simulink model "c00010M_harness"  (R2018a)
settings: Solver=ode3  StartTime=0.0  StopTime=10.0  RelTol=1e-3  EnableMultiTasking=on
undefined symbols (not defined in the file): b, DiscIntNeverNeededParam, J, K, L, PosMinimaW3, R, sigbuilder_block
(part 1 of 4)
settings Model: Creator=aarrieta  LastModifiedBy=umarkiegi
settings DataIOCC: LimitDataPoints=on  SaveFormat=Array
settings OptimizationCC: LifeSpan=inf
settings DebuggingCC: UnderspecifiedInitializationDetection=Classic  MergeDetectMultiDrivingBlocksExec=none  SolverPrmCheckMsg=warning  StateNameClashWarn=warning  SFUnexpectedBacktrackingDiag=warning  SFNoUnconditionalDefaultTransitionDiag=warning  SFExecutionAtInitializationDiag=none
settings HardwareCC: ProdBitPerPointer=32  ProdBitPerSizeT=32  ProdBitPerPtrDiffT=32  ProdLargestAtomicFloat=None  ProdIntDivRoundTo=Undefined  ProdEndianess=Unspecified  ProdWordSize=32  ProdHWDeviceType=32-bit Generic
settings ModelReferenceCC: PropagateSignalLabelsOutOfModel=off
settings CodeAppCC: StateflowObjectComments=on
settings GRTTargetCC: TargetLangStandard=C89/C90 (ANSI)  GeneratePreprocessorConditionals=Disable all
settings ConfigComp: CovMetricSettings=dw  CovHtmlReporting=on  CovSaveCumulativeToWorkspaceVar=on  CovSaveSingleToWorkspaceVar=on  CovExternalEMLEnable=off  DVMaxTestCaseSteps=20  DVTestSuiteOptimization=CombinedObjectives (Nonlinear Extended)  DVDetectFloatOverflow=off

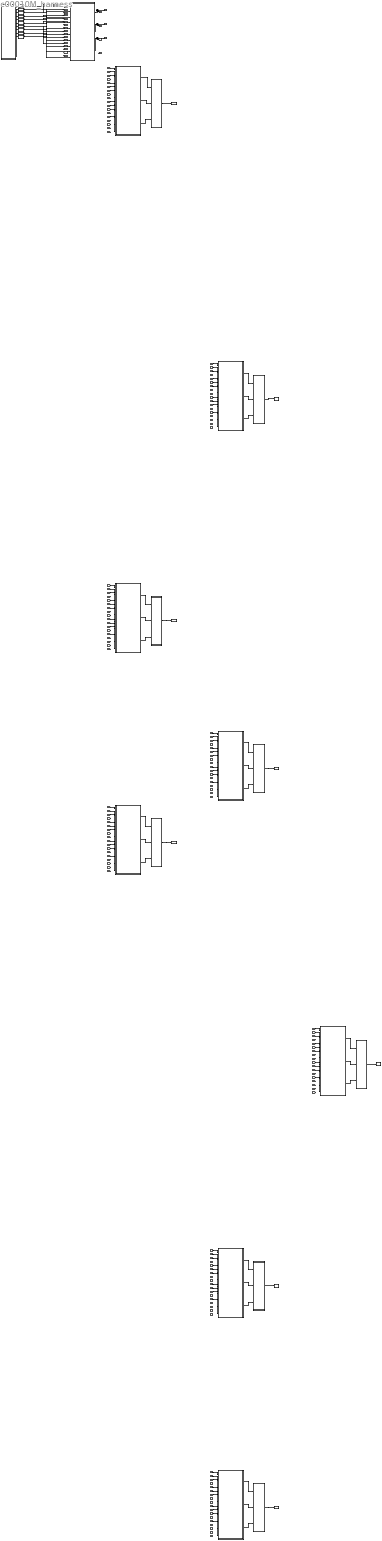
== system c00010M_harness ==
  CPSUT : Subsystem
  Eval : Subsystem
  Eval10 : Subsystem
  Eval24 : Subsystem
  Eval29 : Subsystem
  Eval36 : Subsystem
  Eval39 : Subsystem
  Eval53 : Subsystem
  Eval7 : Subsystem
  Inputs : Subsystem  Tag=STV Subsys  LoadFcn=sigbuilder_block('load');  StartFcn=sigbuilder_block('start');  StopFcn=sigbuilder_block('stop');  ClipboardFcn=sigbuilder_block('clipboard');  mask(Sigbuilder block){tuvar=[0:10]}
      mask init:
      | if ~strcmp(get_param(bdroot(gcb),'SimulationStatus'),'stopped'),tuvar = sigbuilder_block('maskInit'); end
      settings: CopyFcn=sigbuilder_block('copy');  DeleteFcn=sigbuilder_block('delete');  ModelCloseFcn=sigbuilder_block('modelClose');  PreSaveFcn=sigbuilder_block('preSave');  PauseFcn=sigbuilder_block('pause');  ContinueFcn=sigbuilder_block('continue');  NameChangeFcn=sigbuilder_block('namechange');  OpenFcn=sigbuilder_block('open');  CloseFcn=sigbuilder_block('close');
      mask Display: plot(0, 0, 100, 100,[2, 2, 32, 32, 2], [68, 8, 8, 68, 68],[32, 2], [38, 38], [32, 19, 2],[53, 60, 44], [32, 17, 17, 2],[16, 16, 31, 31]);txt = getActiveGroup(gcbh);text(2, 100, txt,'verticalAlignment', 'top');
  M001 : Subsystem
  M008 : Subsystem
  M011 : Subsystem
  M025 : Subsystem
  M030 : Subsystem
  M037 : Subsystem
  M040 : Subsystem
  M054 : Subsystem
  To Workspace : ToWorkspace  VariableName=mutant001  SampleTime=-1
  To Workspace10 : ToWorkspace  VariableName=mutant011  SampleTime=-1
  To Workspace24 : ToWorkspace  VariableName=mutant025  SampleTime=-1
  To Workspace29 : ToWorkspace  VariableName=mutant030  SampleTime=-1
  To Workspace36 : ToWorkspace  VariableName=mutant037  SampleTime=-1
  To Workspace39 : ToWorkspace  VariableName=mutant040  SampleTime=-1
  To Workspace53 : ToWorkspace  VariableName=mutant054  SampleTime=-1
  To Workspace7 : ToWorkspace  VariableName=mutant008  SampleTime=-1
  dtc_DW1 : DataTypeConversion
  dtc_DW2 : DataTypeConversion
  dtc_DW3 : DataTypeConversion
  dtc_LD : DataTypeConversion
  dtc_O1 : DataTypeConversion
  dtc_O2 : DataTypeConversion
  dtc_O3 : DataTypeConversion
  dtc_P1W2 : DataTypeConversion
  dtc_P1W3 : DataTypeConversion
  dtc_P2W3 : DataTypeConversion
  W1Pos : Outport
  W2Pos : Outport  Port=2
  W3Pos : Outport  Port=3
  tag scope: out1=global, out2=global, out3=global, out4=global
  wires:
  CPSUT/2(W2Pos) -> [out2], W2Pos/1
  CPSUT/3(W3Pos) -> W3Pos/1, [out3]
  [in1] -> M001/1(DW1)
  [in2] -> M001/2(DW2)
  [in3] -> M001/3(DW3)
  [in5] -> M001/4(P1W2)
  [in6] -> M001/5(P2W3)
  [in7] -> M001/6(P1W3)
  [in10] -> M001/7(O1)
  [in11] -> M001/8(O2)
  [in12] -> M001/9(O3)
  [in14] -> M001/10(LD)
  CPSUT/1(W1Pos) -> [out1], W1Pos/1
  M001/1(W1Pos) -> Eval/1(In1)
  M001/2(W2Pos) -> Eval/2(In2)
  M001/3(W3Pos) -> Eval/3(In3)
  Eval/1(Out1) -> To Workspace/1
  [in1] -> M008/1(DW1)
  [in2] -> M008/2(DW2)
  [in3] -> M008/3(DW3)
  [in5] -> M008/4(P1W2)
  [in6] -> M008/5(P2W3)
  [in7] -> M008/6(P1W3)
  [in10] -> M008/7(O1)
  [in11] -> M008/8(O2)
  [in12] -> M008/9(O3)
  [in14] -> M008/10(LD)
  M008/1(W1Pos) -> Eval7/1(In1)
  M008/2(W2Pos) -> Eval7/2(In2)
  M008/3(W3Pos) -> Eval7/3(In3)
  Eval7/1(Out1) -> To Workspace7/1
  [in1] -> M011/1(DW1)
  [in2] -> M011/2(DW2)
  [in3] -> M011/3(DW3)
  [in5] -> M011/4(P1W2)
  [in6] -> M011/5(P2W3)
  [in7] -> M011/6(P1W3)
  [in10] -> M011/7(O1)
  [in11] -> M011/8(O2)
  [in12] -> M011/9(O3)
  [in14] -> M011/10(LD)
  M011/1(W1Pos) -> Eval10/1(In1)
  M011/2(W2Pos) -> Eval10/2(In2)
  M011/3(W3Pos) -> Eval10/3(In3)
  Eval10/1(Out1) -> To Workspace10/1
  [in1] -> M025/1(DW1)
  [in2] -> M025/2(DW2)
  [in3] -> M025/3(DW3)
  [in5] -> M025/4(P1W2)
  [in6] -> M025/5(P2W3)
  [in7] -> M025/6(P1W3)
  [in10] -> M025/7(O1)
  [in11] -> M025/8(O2)
  [in12] -> M025/9(O3)
  [in14] -> M025/10(LD)
  M025/1(W1Pos) -> Eval24/1(In1)
  M025/2(W2Pos) -> Eval24/2(In2)
  M025/3(W3Pos) -> Eval24/3(In3)
  Eval24/1(Out1) -> To Workspace24/1
  [in1] -> M030/1(DW1)
  [in2] -> M030/2(DW2)
  [in3] -> M030/3(DW3)
  [in5] -> M030/4(P1W2)
  [in6] -> M030/5(P2W3)
  [in7] -> M030/6(P1W3)
  [in10] -> M030/7(O1)
  [in11] -> M030/8(O2)
  [in12] -> M030/9(O3)
  [in14] -> M030/10(LD)
  M030/1(W1Pos) -> Eval29/1(In1)
  M030/2(W2Pos) -> Eval29/2(In2)
  M030/3(W3Pos) -> Eval29/3(In3)
  Eval29/1(Out1) -> To Workspace29/1
  [in1] -> M037/1(DW1)
  [in2] -> M037/2(DW2)
  [in3] -> M037/3(DW3)
  [in5] -> M037/4(P1W2)
  [in6] -> M037/5(P2W3)
  [in7] -> M037/6(P1W3)
  [in10] -> M037/7(O1)
  [in11] -> M037/8(O2)
  [in12] -> M037/9(O3)
  [in14] -> M037/10(LD)
  M037/1(W1Pos) -> Eval36/1(In1)
  M037/2(W2Pos) -> Eval36/2(In2)
  M037/3(W3Pos) -> Eval36/3(In3)
  Eval36/1(Out1) -> To Workspace36/1
  [in1] -> M040/1(DW1)
  [in2] -> M040/2(DW2)
  [in3] -> M040/3(DW3)
  [in5] -> M040/4(P1W2)
  [in6] -> M040/5(P2W3)
  [in7] -> M040/6(P1W3)
  [in10] -> M040/7(O1)
  [in11] -> M040/8(O2)
  [in12] -> M040/9(O3)
  [in14] -> M040/10(LD)
  M040/1(W1Pos) -> Eval39/1(In1)
  M040/2(W2Pos) -> Eval39/2(In2)
  M040/3(W3Pos) -> Eval39/3(In3)
  Eval39/1(Out1) -> To Workspace39/1
  [in1] -> M054/1(DW1)
  [in2] -> M054/2(DW2)
  [in3] -> M054/3(DW3)
  [in5] -> M054/4(P1W2)
  [in6] -> M054/5(P2W3)
  [in7] -> M054/6(P1W3)
  [in10] -> M054/7(O1)
  [in11] -> M054/8(O2)
  [in12] -> M054/9(O3)
  [in14] -> M054/10(LD)
  M054/1(W1Pos) -> Eval53/1(In1)
  M054/2(W2Pos) -> Eval53/2(In2)
  M054/3(W3Pos) -> Eval53/3(In3)
  Eval53/1(Out1) -> To Workspace53/1
  Inputs/1(DW1) -> dtc_DW1/1
  dtc_DW1/1 -> CPSUT/1(DW1), [in1]
  Inputs/2(DW2) -> dtc_DW2/1
  dtc_DW2/1 -> CPSUT/2(DW2), [in2]
  Inputs/3(DW3) -> dtc_DW3/1
  dtc_DW3/1 -> CPSUT/3(DW3), [in3]
  Inputs/4(P1W2) -> dtc_P1W2/1
  dtc_P1W2/1 -> CPSUT/4(P1W2), [in5]
  Inputs/5(P2W3) -> dtc_P2W3/1
  dtc_P2W3/1 -> CPSUT/5(P2W3), [in6]
  Inputs/6(P1W3) -> dtc_P1W3/1
  dtc_P1W3/1 -> CPSUT/6(P1W3), [in7]
  Inputs/7(O1) -> dtc_O1/1
  dtc_O1/1 -> CPSUT/7(O1), [in10]
  Inputs/8(O2) -> dtc_O2/1
  dtc_O2/1 -> CPSUT/8(O2), [in11]
  Inputs/9(O3) -> dtc_O3/1
  dtc_O3/1 -> CPSUT/9(O3), [in12]
  Inputs/10(LD) -> dtc_LD/1
  dtc_LD/1 -> CPSUT/10(LD), [in14]

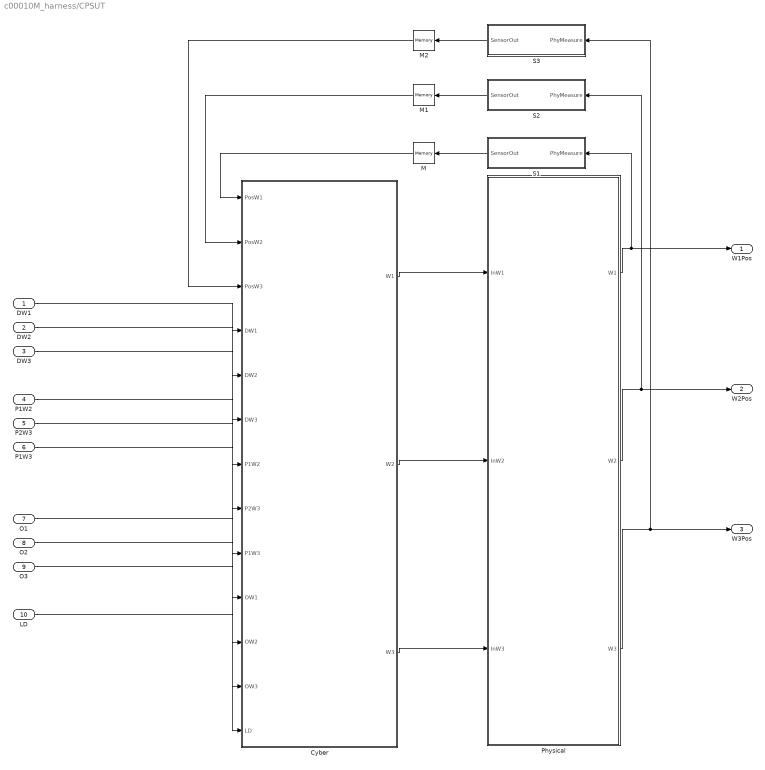
== system c00010M_harness/CPSUT ==
  DW1 : Inport  OutMin=0  OutMax=4  OutDataTypeStr=int8
  DW2 : Inport  Port=2  OutMin=0  OutMax=4  OutDataTypeStr=int8
  DW3 : Inport  Port=3  OutMin=0  OutMax=4  OutDataTypeStr=int8
  P1W2 : Inport  Port=4  OutMin=0  OutMax=4  OutDataTypeStr=int8
  P2W3 : Inport  Port=5  OutMin=0  OutMax=4  OutDataTypeStr=int8
  P1W3 : Inport  Port=6  OutMin=0  OutMax=4  OutDataTypeStr=int8
  O1 : Inport  Port=7  OutDataTypeStr=boolean
  O2 : Inport  Port=8  OutDataTypeStr=boolean
  O3 : Inport  Port=9  OutDataTypeStr=boolean
  LD : Inport  Port=10  OutDataTypeStr=boolean
  Cyber : Subsystem
  M : Memory
  M1 : Memory
  M2 : Memory
  Physical : Subsystem
  S1 : Subsystem
  S2 : Subsystem
  S3 : Subsystem
  W1Pos : Outport
  W2Pos : Outport  Port=2
  W3Pos : Outport  Port=3
  wires:
  P2W3/1 -> Cyber/8(P2W3)
  S1/1(SensorOut) -> M/1
  Physical/1(W1) -> W1Pos/1, S1/1(PhyMeasure)
  S3/1(SensorOut) -> M2/1
  O2/1 -> Cyber/11(OW2)
  Cyber/3(W3) -> Physical/3(InW3)
  LD/1 -> Cyber/13(LD)
  O1/1 -> Cyber/10(OW1)
  Cyber/1(W1) -> Physical/1(InW1)
  Cyber/2(W2) -> Physical/2(InW2)
  M2/1 -> Cyber/3(PosW3)
  P1W2/1 -> Cyber/7(P1W2)
  O3/1 -> Cyber/12(OW3)
  P1W3/1 -> Cyber/9(P1W3)
  DW3/1 -> Cyber/6(DW3)
  M1/1 -> Cyber/2(PosW2)
  Physical/3(W3) -> W3Pos/1, S3/1(PhyMeasure)
  M/1 -> Cyber/1(PosW1)
  DW1/1 -> Cyber/4(DW1)
  Physical/2(W2) -> W2Pos/1, S2/1(PhyMeasure)
  S2/1(SensorOut) -> M1/1
  DW2/1 -> Cyber/5(DW2)

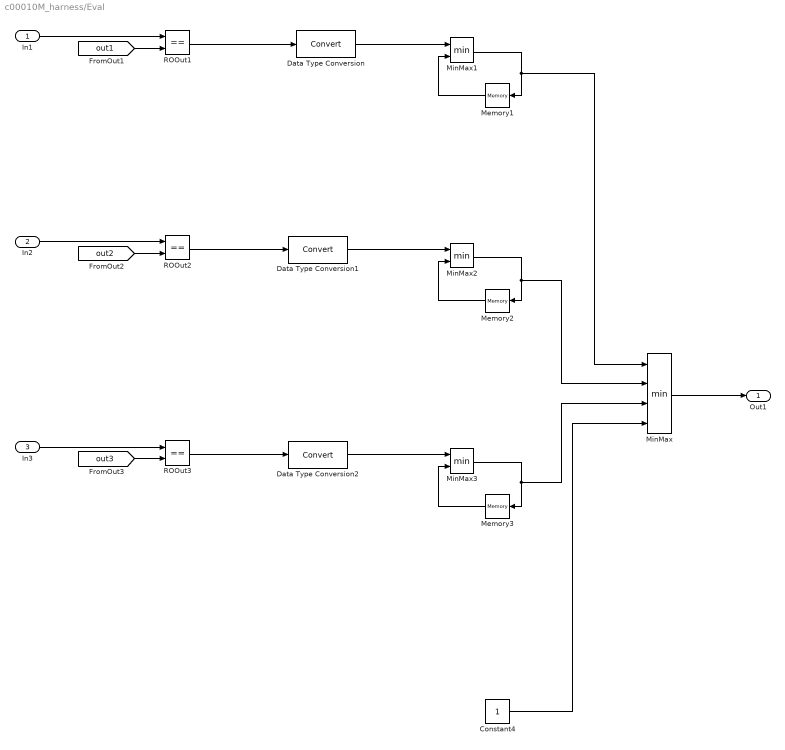
== system c00010M_harness/Eval ==
  In1 : Inport
  In2 : Inport  Port=2
  In3 : Inport  Port=3
  Constant4 : Constant
  Data Type Conversion : DataTypeConversion
  Data Type Conversion1 : DataTypeConversion
  Data Type Conversion2 : DataTypeConversion
  Memory1 : Memory  InitialCondition=1
  Memory2 : Memory  InitialCondition=1
  Memory3 : Memory  InitialCondition=1
  MinMax : MinMax  Inputs=4
  MinMax1 : MinMax  Inputs=2
  MinMax2 : MinMax  Inputs=2
  MinMax3 : MinMax  Inputs=2
  ROOut1 : RelationalOperator  Operator===  OutDataTypeStr=boolean  RndMeth=Simplest
  ROOut2 : RelationalOperator  Operator===  OutDataTypeStr=boolean  RndMeth=Simplest
  ROOut3 : RelationalOperator  Operator===  OutDataTypeStr=boolean  RndMeth=Simplest
  Out1 : Outport
  wires:
  MinMax/1 -> Out1/1
  [out3] -> ROOut3/2
  In3/1 -> ROOut3/1
  [out1] -> ROOut1/2
  In2/1 -> ROOut2/1
  In1/1 -> ROOut1/1
  [out2] -> ROOut2/2
  Memory1/1 -> MinMax1/2
  MinMax3/1 -> MinMax/3, Memory3/1
  ROOut3/1 -> Data Type Conversion2/1
  ROOut2/1 -> Data Type Conversion1/1
  Memory3/1 -> MinMax3/2
  Memory2/1 -> MinMax2/2
  ROOut1/1 -> Data Type Conversion/1
  MinMax2/1 -> MinMax/2, Memory2/1
  MinMax1/1 -> MinMax/1, Memory1/1
  Data Type Conversion/1 -> MinMax1/1
  Data Type Conversion1/1 -> MinMax2/1
  Data Type Conversion2/1 -> MinMax3/1
  Constant4/1 -> MinMax/4

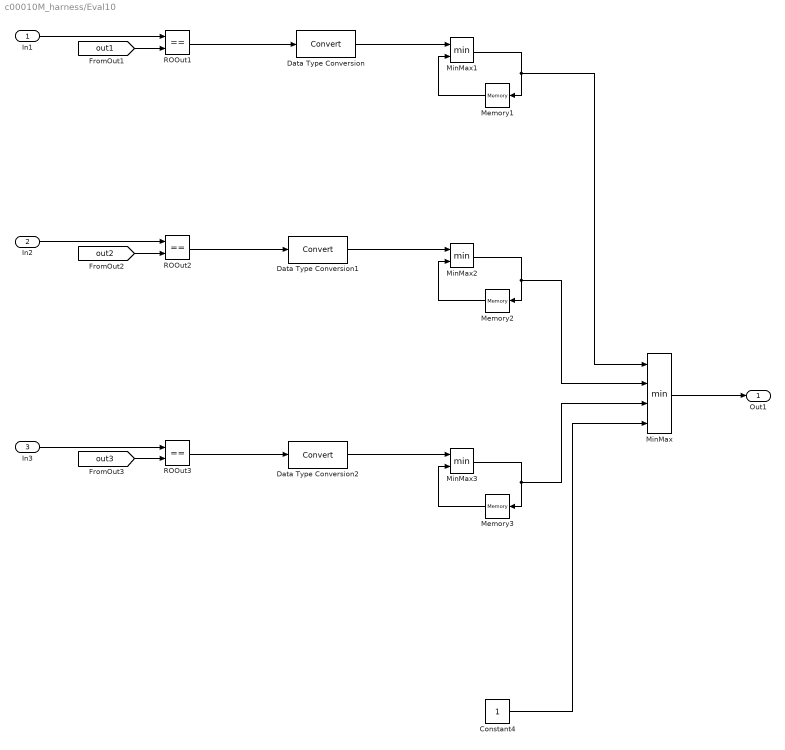
== system c00010M_harness/Eval10 ==
  In1 : Inport
  In2 : Inport  Port=2
  In3 : Inport  Port=3
  Constant4 : Constant
  Data Type Conversion : DataTypeConversion
  Data Type Conversion1 : DataTypeConversion
  Data Type Conversion2 : DataTypeConversion
  Memory1 : Memory  InitialCondition=1
  Memory2 : Memory  InitialCondition=1
  Memory3 : Memory  InitialCondition=1
  MinMax : MinMax  Inputs=4
  MinMax1 : MinMax  Inputs=2
  MinMax2 : MinMax  Inputs=2
  MinMax3 : MinMax  Inputs=2
  ROOut1 : RelationalOperator  Operator===  OutDataTypeStr=boolean  RndMeth=Simplest
  ROOut2 : RelationalOperator  Operator===  OutDataTypeStr=boolean  RndMeth=Simplest
  ROOut3 : RelationalOperator  Operator===  OutDataTypeStr=boolean  RndMeth=Simplest
  Out1 : Outport
  wires:
  Data Type Conversion2/1 -> MinMax3/1
  Data Type Conversion1/1 -> MinMax2/1
  Data Type Conversion/1 -> MinMax1/1
  MinMax1/1 -> Memory1/1, MinMax/1
  MinMax2/1 -> Memory2/1, MinMax/2
  ROOut1/1 -> Data Type Conversion/1
  Memory2/1 -> MinMax2/2
  Memory3/1 -> MinMax3/2
  ROOut2/1 -> Data Type Conversion1/1
  ROOut3/1 -> Data Type Conversion2/1
  MinMax3/1 -> Memory3/1, MinMax/3
  Memory1/1 -> MinMax1/2
  [out2] -> ROOut2/2
  In1/1 -> ROOut1/1
  In2/1 -> ROOut2/1
  [out1] -> ROOut1/2
  In3/1 -> ROOut3/1
  [out3] -> ROOut3/2
  MinMax/1 -> Out1/1
  Constant4/1 -> MinMax/4

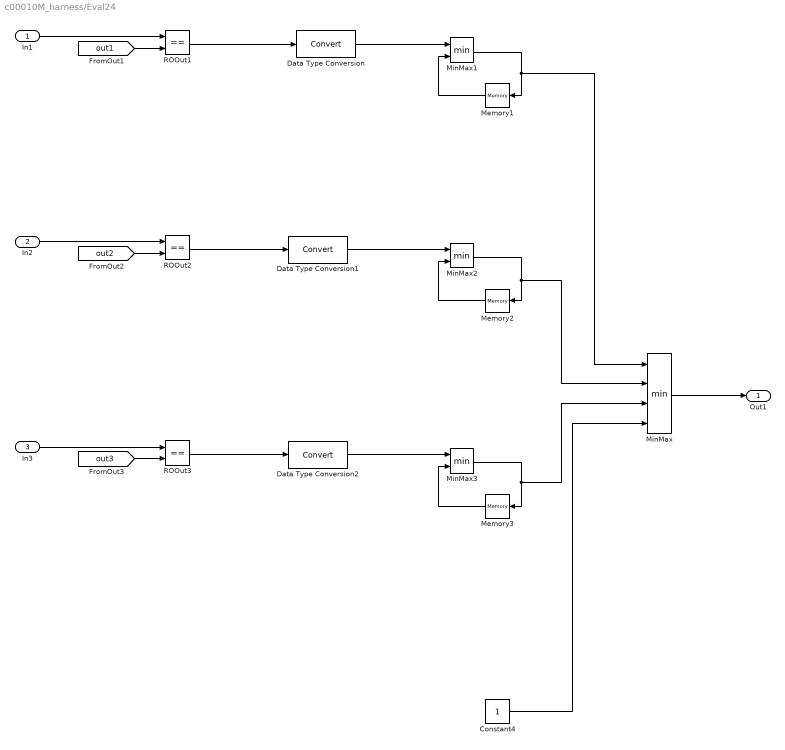
== system c00010M_harness/Eval24 ==
  In1 : Inport
  In2 : Inport  Port=2
  In3 : Inport  Port=3
  Constant4 : Constant
  Data Type Conversion : DataTypeConversion
  Data Type Conversion1 : DataTypeConversion
  Data Type Conversion2 : DataTypeConversion
  Memory1 : Memory  InitialCondition=1
  Memory2 : Memory  InitialCondition=1
  Memory3 : Memory  InitialCondition=1
  MinMax : MinMax  Inputs=4
  MinMax1 : MinMax  Inputs=2
  MinMax2 : MinMax  Inputs=2
  MinMax3 : MinMax  Inputs=2
  ROOut1 : RelationalOperator  Operator===  OutDataTypeStr=boolean  RndMeth=Simplest
  ROOut2 : RelationalOperator  Operator===  OutDataTypeStr=boolean  RndMeth=Simplest
  ROOut3 : RelationalOperator  Operator===  OutDataTypeStr=boolean  RndMeth=Simplest
  Out1 : Outport
  wires:
  Data Type Conversion2/1 -> MinMax3/1
  Data Type Conversion1/1 -> MinMax2/1
  Data Type Conversion/1 -> MinMax1/1
  MinMax1/1 -> Memory1/1, MinMax/1
  MinMax2/1 -> Memory2/1, MinMax/2
  ROOut1/1 -> Data Type Conversion/1
  Memory2/1 -> MinMax2/2
  Memory3/1 -> MinMax3/2
  ROOut2/1 -> Data Type Conversion1/1
  ROOut3/1 -> Data Type Conversion2/1
  MinMax3/1 -> Memory3/1, MinMax/3
  Memory1/1 -> MinMax1/2
  [out2] -> ROOut2/2
  In1/1 -> ROOut1/1
  In2/1 -> ROOut2/1
  [out1] -> ROOut1/2
  In3/1 -> ROOut3/1
  [out3] -> ROOut3/2
  MinMax/1 -> Out1/1
  Constant4/1 -> MinMax/4

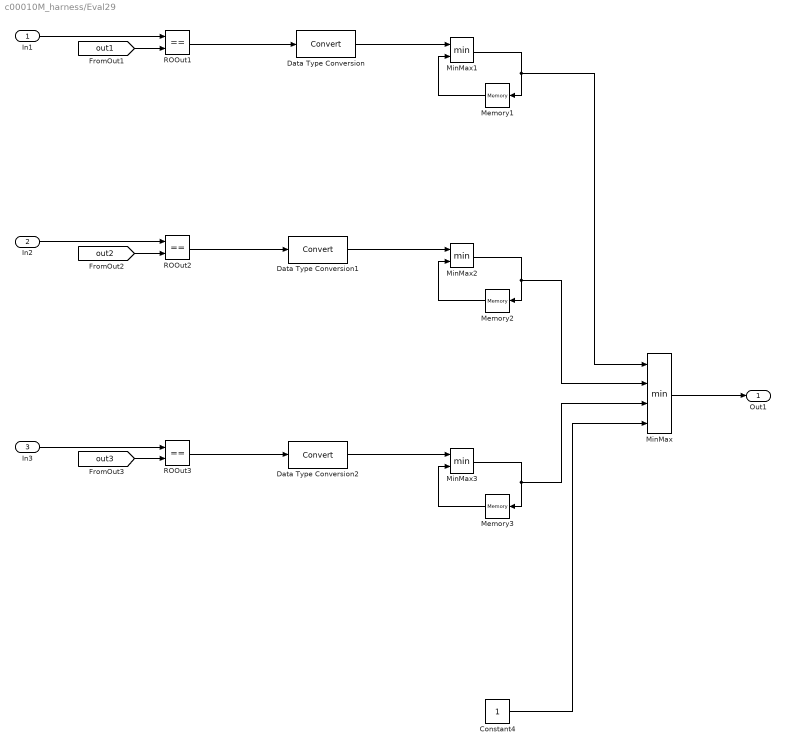
== system c00010M_harness/Eval29 ==
  In1 : Inport
  In2 : Inport  Port=2
  In3 : Inport  Port=3
  Constant4 : Constant
  Data Type Conversion : DataTypeConversion
  Data Type Conversion1 : DataTypeConversion
  Data Type Conversion2 : DataTypeConversion
  Memory1 : Memory  InitialCondition=1
  Memory2 : Memory  InitialCondition=1
  Memory3 : Memory  InitialCondition=1
  MinMax : MinMax  Inputs=4
  MinMax1 : MinMax  Inputs=2
  MinMax2 : MinMax  Inputs=2
  MinMax3 : MinMax  Inputs=2
  ROOut1 : RelationalOperator  Operator===  OutDataTypeStr=boolean  RndMeth=Simplest
  ROOut2 : RelationalOperator  Operator===  OutDataTypeStr=boolean  RndMeth=Simplest
  ROOut3 : RelationalOperator  Operator===  OutDataTypeStr=boolean  RndMeth=Simplest
  Out1 : Outport
  wires:
  Data Type Conversion2/1 -> MinMax3/1
  Data Type Conversion1/1 -> MinMax2/1
  Data Type Conversion/1 -> MinMax1/1
  MinMax1/1 -> Memory1/1, MinMax/1
  MinMax2/1 -> Memory2/1, MinMax/2
  ROOut1/1 -> Data Type Conversion/1
  Memory2/1 -> MinMax2/2
  Memory3/1 -> MinMax3/2
  ROOut2/1 -> Data Type Conversion1/1
  ROOut3/1 -> Data Type Conversion2/1
  MinMax3/1 -> Memory3/1, MinMax/3
  Memory1/1 -> MinMax1/2
  [out2] -> ROOut2/2
  In1/1 -> ROOut1/1
  In2/1 -> ROOut2/1
  [out1] -> ROOut1/2
  In3/1 -> ROOut3/1
  [out3] -> ROOut3/2
  MinMax/1 -> Out1/1
  Constant4/1 -> MinMax/4

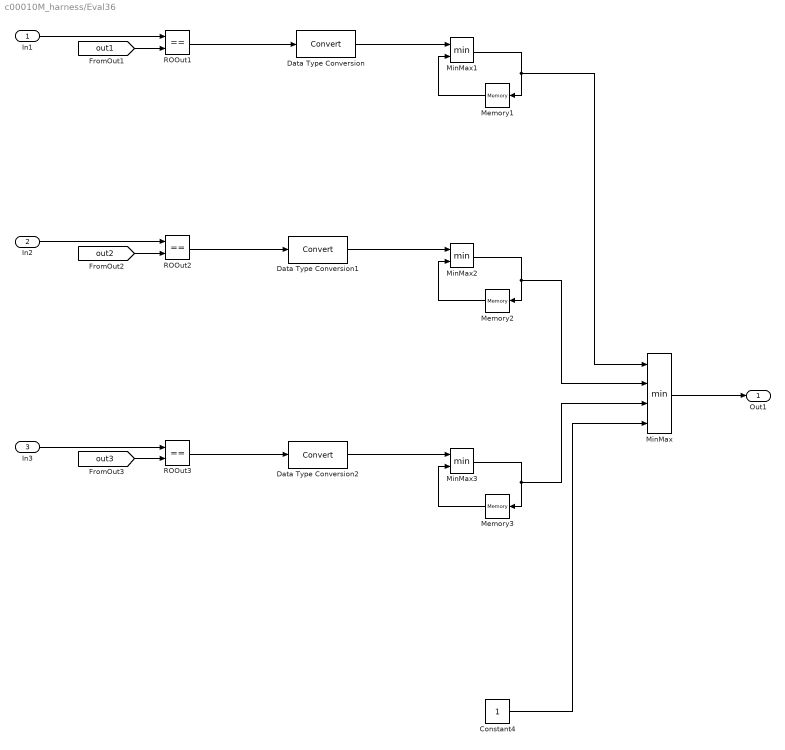
== system c00010M_harness/Eval36 ==
  In1 : Inport
  In2 : Inport  Port=2
  In3 : Inport  Port=3
  Constant4 : Constant
  Data Type Conversion : DataTypeConversion
  Data Type Conversion1 : DataTypeConversion
  Data Type Conversion2 : DataTypeConversion
  Memory1 : Memory  InitialCondition=1
  Memory2 : Memory  InitialCondition=1
  Memory3 : Memory  InitialCondition=1
  MinMax : MinMax  Inputs=4
  MinMax1 : MinMax  Inputs=2
  MinMax2 : MinMax  Inputs=2
  MinMax3 : MinMax  Inputs=2
  ROOut1 : RelationalOperator  Operator===  OutDataTypeStr=boolean  RndMeth=Simplest
  ROOut2 : RelationalOperator  Operator===  OutDataTypeStr=boolean  RndMeth=Simplest
  ROOut3 : RelationalOperator  Operator===  OutDataTypeStr=boolean  RndMeth=Simplest
  Out1 : Outport
  wires:
  Data Type Conversion2/1 -> MinMax3/1
  Data Type Conversion1/1 -> MinMax2/1
  Data Type Conversion/1 -> MinMax1/1
  MinMax1/1 -> Memory1/1, MinMax/1
  MinMax2/1 -> Memory2/1, MinMax/2
  ROOut1/1 -> Data Type Conversion/1
  Memory2/1 -> MinMax2/2
  Memory3/1 -> MinMax3/2
  ROOut2/1 -> Data Type Conversion1/1
  ROOut3/1 -> Data Type Conversion2/1
  MinMax3/1 -> Memory3/1, MinMax/3
  Memory1/1 -> MinMax1/2
  [out2] -> ROOut2/2
  In1/1 -> ROOut1/1
  In2/1 -> ROOut2/1
  [out1] -> ROOut1/2
  In3/1 -> ROOut3/1
  [out3] -> ROOut3/2
  MinMax/1 -> Out1/1
  Constant4/1 -> MinMax/4

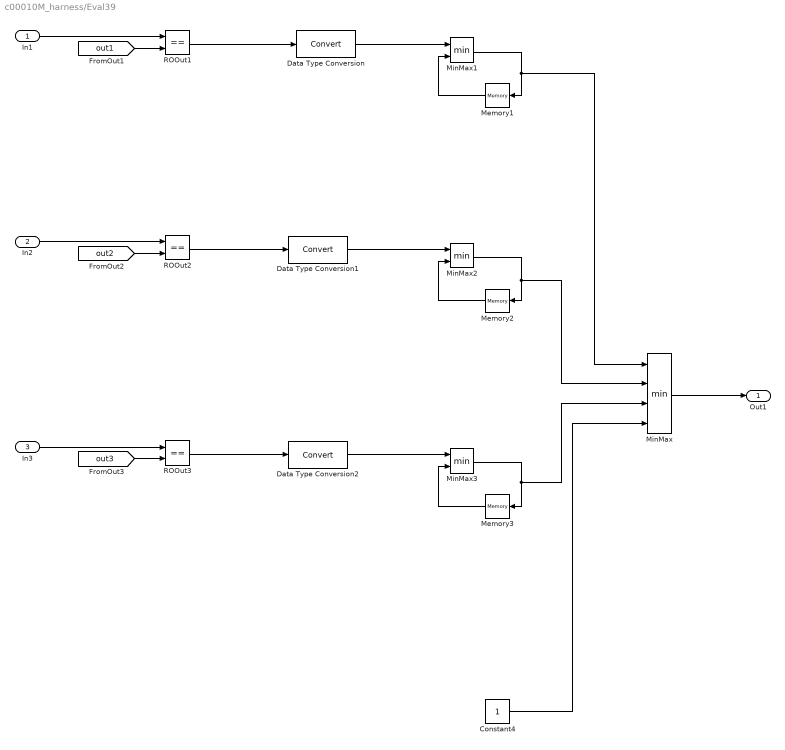
== system c00010M_harness/Eval39 ==
  In1 : Inport
  In2 : Inport  Port=2
  In3 : Inport  Port=3
  Constant4 : Constant
  Data Type Conversion : DataTypeConversion
  Data Type Conversion1 : DataTypeConversion
  Data Type Conversion2 : DataTypeConversion
  Memory1 : Memory  InitialCondition=1
  Memory2 : Memory  InitialCondition=1
  Memory3 : Memory  InitialCondition=1
  MinMax : MinMax  Inputs=4
  MinMax1 : MinMax  Inputs=2
  MinMax2 : MinMax  Inputs=2
  MinMax3 : MinMax  Inputs=2
  ROOut1 : RelationalOperator  Operator===  OutDataTypeStr=boolean  RndMeth=Simplest
  ROOut2 : RelationalOperator  Operator===  OutDataTypeStr=boolean  RndMeth=Simplest
  ROOut3 : RelationalOperator  Operator===  OutDataTypeStr=boolean  RndMeth=Simplest
  Out1 : Outport
  wires:
  Data Type Conversion2/1 -> MinMax3/1
  Data Type Conversion1/1 -> MinMax2/1
  Data Type Conversion/1 -> MinMax1/1
  MinMax1/1 -> Memory1/1, MinMax/1
  MinMax2/1 -> Memory2/1, MinMax/2
  ROOut1/1 -> Data Type Conversion/1
  Memory2/1 -> MinMax2/2
  Memory3/1 -> MinMax3/2
  ROOut2/1 -> Data Type Conversion1/1
  ROOut3/1 -> Data Type Conversion2/1
  MinMax3/1 -> Memory3/1, MinMax/3
  Memory1/1 -> MinMax1/2
  [out2] -> ROOut2/2
  In1/1 -> ROOut1/1
  In2/1 -> ROOut2/1
  [out1] -> ROOut1/2
  In3/1 -> ROOut3/1
  [out3] -> ROOut3/2
  MinMax/1 -> Out1/1
  Constant4/1 -> MinMax/4

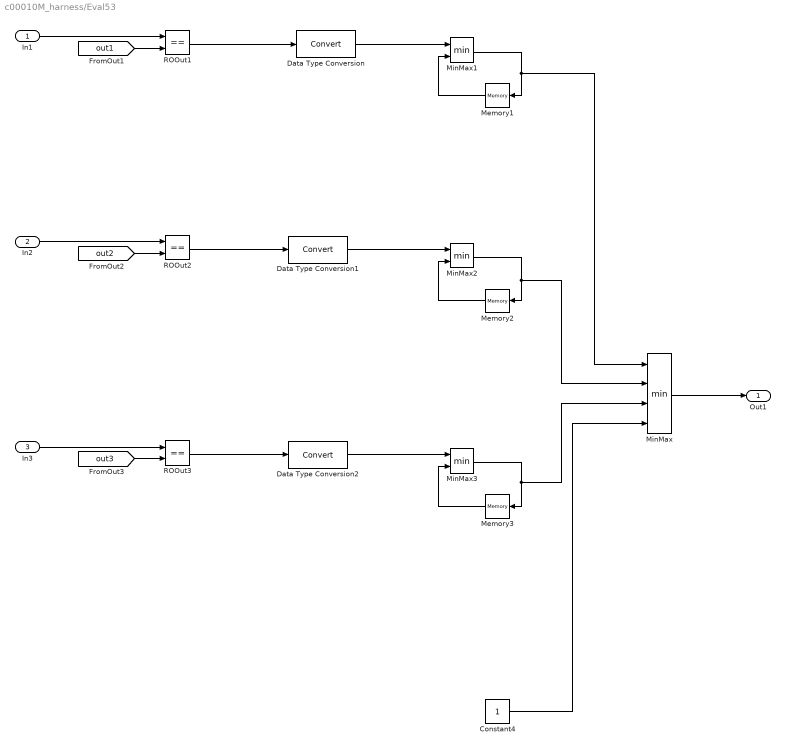
== system c00010M_harness/Eval53 ==
  In1 : Inport
  In2 : Inport  Port=2
  In3 : Inport  Port=3
  Constant4 : Constant
  Data Type Conversion : DataTypeConversion
  Data Type Conversion1 : DataTypeConversion
  Data Type Conversion2 : DataTypeConversion
  Memory1 : Memory  InitialCondition=1
  Memory2 : Memory  InitialCondition=1
  Memory3 : Memory  InitialCondition=1
  MinMax : MinMax  Inputs=4
  MinMax1 : MinMax  Inputs=2
  MinMax2 : MinMax  Inputs=2
  MinMax3 : MinMax  Inputs=2
  ROOut1 : RelationalOperator  Operator===  OutDataTypeStr=boolean  RndMeth=Simplest
  ROOut2 : RelationalOperator  Operator===  OutDataTypeStr=boolean  RndMeth=Simplest
  ROOut3 : RelationalOperator  Operator===  OutDataTypeStr=boolean  RndMeth=Simplest
  Out1 : Outport
  wires:
  Data Type Conversion2/1 -> MinMax3/1
  Data Type Conversion1/1 -> MinMax2/1
  Data Type Conversion/1 -> MinMax1/1
  MinMax1/1 -> Memory1/1, MinMax/1
  MinMax2/1 -> Memory2/1, MinMax/2
  ROOut1/1 -> Data Type Conversion/1
  Memory2/1 -> MinMax2/2
  Memory3/1 -> MinMax3/2
  ROOut2/1 -> Data Type Conversion1/1
  ROOut3/1 -> Data Type Conversion2/1
  MinMax3/1 -> Memory3/1, MinMax/3
  Memory1/1 -> MinMax1/2
  [out2] -> ROOut2/2
  In1/1 -> ROOut1/1
  In2/1 -> ROOut2/1
  [out1] -> ROOut1/2
  In3/1 -> ROOut3/1
  [out3] -> ROOut3/2
  MinMax/1 -> Out1/1
  Constant4/1 -> MinMax/4

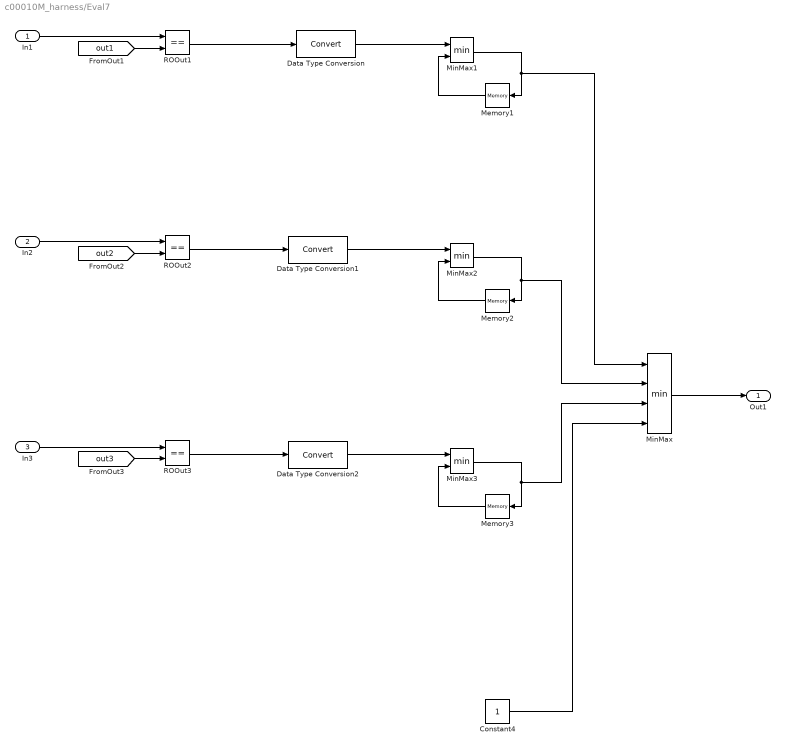
== system c00010M_harness/Eval7 ==
  In1 : Inport
  In2 : Inport  Port=2
  In3 : Inport  Port=3
  Constant4 : Constant
  Data Type Conversion : DataTypeConversion
  Data Type Conversion1 : DataTypeConversion
  Data Type Conversion2 : DataTypeConversion
  Memory1 : Memory  InitialCondition=1
  Memory2 : Memory  InitialCondition=1
  Memory3 : Memory  InitialCondition=1
  MinMax : MinMax  Inputs=4
  MinMax1 : MinMax  Inputs=2
  MinMax2 : MinMax  Inputs=2
  MinMax3 : MinMax  Inputs=2
  ROOut1 : RelationalOperator  Operator===  OutDataTypeStr=boolean  RndMeth=Simplest
  ROOut2 : RelationalOperator  Operator===  OutDataTypeStr=boolean  RndMeth=Simplest
  ROOut3 : RelationalOperator  Operator===  OutDataTypeStr=boolean  RndMeth=Simplest
  Out1 : Outport
  wires:
  Data Type Conversion2/1 -> MinMax3/1
  Data Type Conversion1/1 -> MinMax2/1
  Data Type Conversion/1 -> MinMax1/1
  MinMax1/1 -> Memory1/1, MinMax/1
  MinMax2/1 -> Memory2/1, MinMax/2
  ROOut1/1 -> Data Type Conversion/1
  Memory2/1 -> MinMax2/2
  Memory3/1 -> MinMax3/2
  ROOut2/1 -> Data Type Conversion1/1
  ROOut3/1 -> Data Type Conversion2/1
  MinMax3/1 -> Memory3/1, MinMax/3
  Memory1/1 -> MinMax1/2
  [out2] -> ROOut2/2
  In1/1 -> ROOut1/1
  In2/1 -> ROOut2/1
  [out1] -> ROOut1/2
  In3/1 -> ROOut3/1
  [out3] -> ROOut3/2
  MinMax/1 -> Out1/1
  Constant4/1 -> MinMax/4

== system c00010M_harness/Inputs ==
  Demux : Demux  Tag=STV Demux  Outputs=10
  FromWs : FromWorkspace  Tag=STV FromWs  VariableName=tuvar  SampleTime=0
  DW1 : Outport  Tag=STV Outport
  DW2 : Outport  Tag=STV Outport  Port=2
  DW3 : Outport  Tag=STV Outport  Port=3
  P1W2 : Outport  Tag=STV Outport  Port=4
  P2W3 : Outport  Tag=STV Outport  Port=5
  P1W3 : Outport  Tag=STV Outport  Port=6
  O1 : Outport  Tag=STV Outport  Port=7
  O2 : Outport  Tag=STV Outport  Port=8
  O3 : Outport  Tag=STV Outport  Port=9
  LD : Outport  Tag=STV Outport  Port=10
  wires:
  Demux/10 -> LD/1
  Demux/9 -> O3/1
  Demux/8 -> O2/1
  Demux/7 -> O1/1
  Demux/6 -> P1W3/1
  Demux/5 -> P2W3/1
  Demux/4 -> P1W2/1
  Demux/3 -> DW3/1
  Demux/2 -> DW2/1
  Demux/1 -> DW1/1
  FromWs/1 -> Demux/1

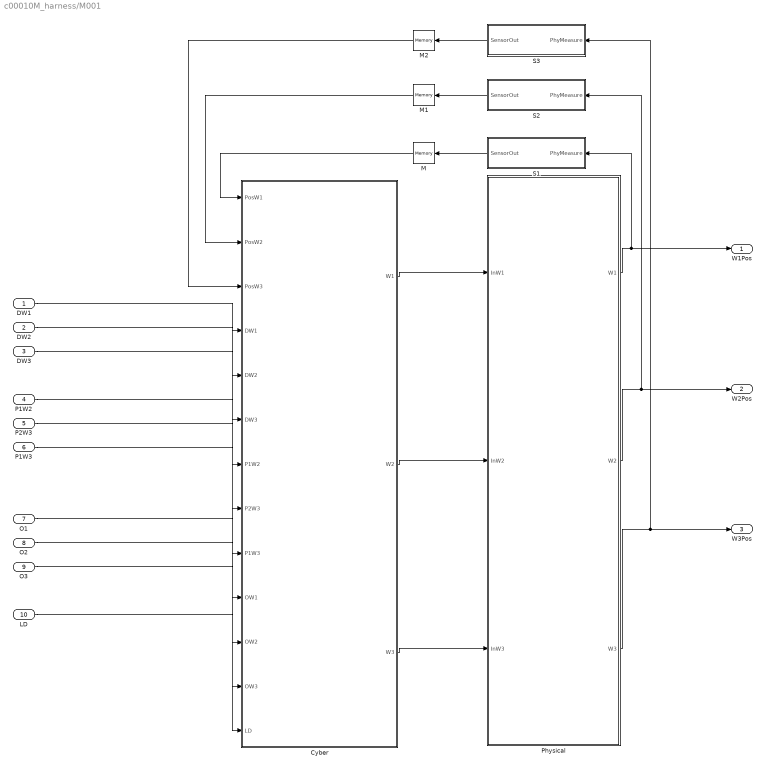
== system c00010M_harness/M001 ==
  DW1 : Inport  OutMin=0  OutMax=4  OutDataTypeStr=int8
  DW2 : Inport  Port=2  OutMin=0  OutMax=4  OutDataTypeStr=int8
  DW3 : Inport  Port=3  OutMin=0  OutMax=4  OutDataTypeStr=int8
  P1W2 : Inport  Port=4  OutMin=0  OutMax=4  OutDataTypeStr=int8
  P2W3 : Inport  Port=5  OutMin=0  OutMax=4  OutDataTypeStr=int8
  P1W3 : Inport  Port=6  OutMin=0  OutMax=4  OutDataTypeStr=int8
  O1 : Inport  Port=7  OutDataTypeStr=boolean
  O2 : Inport  Port=8  OutDataTypeStr=boolean
  O3 : Inport  Port=9  OutDataTypeStr=boolean
  LD : Inport  Port=10  OutDataTypeStr=boolean
  Cyber : Subsystem
  M : Memory
  M1 : Memory
  M2 : Memory
  Physical : Subsystem
  S1 : Subsystem
  S2 : Subsystem
  S3 : Subsystem
  W1Pos : Outport
  W2Pos : Outport  Port=2
  W3Pos : Outport  Port=3
  wires:
  P2W3/1 -> Cyber/8(P2W3)
  S1/1(SensorOut) -> M/1
  Physical/1(W1) -> W1Pos/1, S1/1(PhyMeasure)
  S3/1(SensorOut) -> M2/1
  O2/1 -> Cyber/11(OW2)
  Cyber/3(W3) -> Physical/3(InW3)
  LD/1 -> Cyber/13(LD)
  O1/1 -> Cyber/10(OW1)
  Cyber/1(W1) -> Physical/1(InW1)
  Cyber/2(W2) -> Physical/2(InW2)
  M2/1 -> Cyber/3(PosW3)
  P1W2/1 -> Cyber/7(P1W2)
  O3/1 -> Cyber/12(OW3)
  P1W3/1 -> Cyber/9(P1W3)
  DW3/1 -> Cyber/6(DW3)
  M1/1 -> Cyber/2(PosW2)
  Physical/3(W3) -> W3Pos/1, S3/1(PhyMeasure)
  M/1 -> Cyber/1(PosW1)
  DW1/1 -> Cyber/4(DW1)
  Physical/2(W2) -> W2Pos/1, S2/1(PhyMeasure)
  S2/1(SensorOut) -> M1/1
  DW2/1 -> Cyber/5(DW2)

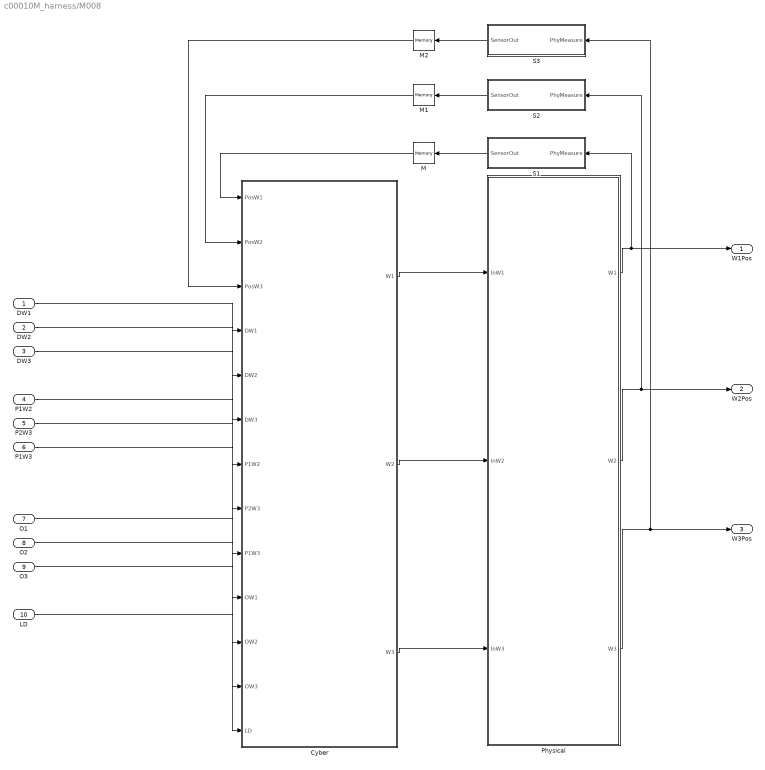
== system c00010M_harness/M008 ==
  DW1 : Inport  OutMin=0  OutMax=4  OutDataTypeStr=int8
  DW2 : Inport  Port=2  OutMin=0  OutMax=4  OutDataTypeStr=int8
  DW3 : Inport  Port=3  OutMin=0  OutMax=4  OutDataTypeStr=int8
  P1W2 : Inport  Port=4  OutMin=0  OutMax=4  OutDataTypeStr=int8
  P2W3 : Inport  Port=5  OutMin=0  OutMax=4  OutDataTypeStr=int8
  P1W3 : Inport  Port=6  OutMin=0  OutMax=4  OutDataTypeStr=int8
  O1 : Inport  Port=7  OutDataTypeStr=boolean
  O2 : Inport  Port=8  OutDataTypeStr=boolean
  O3 : Inport  Port=9  OutDataTypeStr=boolean
  LD : Inport  Port=10  OutDataTypeStr=boolean
  Cyber : Subsystem
  M : Memory
  M1 : Memory
  M2 : Memory
  Physical : Subsystem
  S1 : Subsystem
  S2 : Subsystem
  S3 : Subsystem
  W1Pos : Outport
  W2Pos : Outport  Port=2
  W3Pos : Outport  Port=3
  wires:
  DW2/1 -> Cyber/5(DW2)
  S2/1(SensorOut) -> M1/1
  Physical/2(W2) -> S2/1(PhyMeasure), W2Pos/1
  DW1/1 -> Cyber/4(DW1)
  M/1 -> Cyber/1(PosW1)
  Physical/3(W3) -> S3/1(PhyMeasure), W3Pos/1
  M1/1 -> Cyber/2(PosW2)
  DW3/1 -> Cyber/6(DW3)
  P1W3/1 -> Cyber/9(P1W3)
  O3/1 -> Cyber/12(OW3)
  P1W2/1 -> Cyber/7(P1W2)
  M2/1 -> Cyber/3(PosW3)
  Cyber/2(W2) -> Physical/2(InW2)
  Cyber/1(W1) -> Physical/1(InW1)
  O1/1 -> Cyber/10(OW1)
  LD/1 -> Cyber/13(LD)
  Cyber/3(W3) -> Physical/3(InW3)
  O2/1 -> Cyber/11(OW2)
  S3/1(SensorOut) -> M2/1
  Physical/1(W1) -> S1/1(PhyMeasure), W1Pos/1
  S1/1(SensorOut) -> M/1
  P2W3/1 -> Cyber/8(P2W3)

== system c00010M_harness/M011 ==
  DW1 : Inport  OutMin=0  OutMax=4  OutDataTypeStr=int8
  DW2 : Inport  Port=2  OutMin=0  OutMax=4  OutDataTypeStr=int8
  DW3 : Inport  Port=3  OutMin=0  OutMax=4  OutDataTypeStr=int8
  P1W2 : Inport  Port=4  OutMin=0  OutMax=4  OutDataTypeStr=int8
  P2W3 : Inport  Port=5  OutMin=0  OutMax=4  OutDataTypeStr=int8
  P1W3 : Inport  Port=6  OutMin=0  OutMax=4  OutDataTypeStr=int8
  O1 : Inport  Port=7  OutDataTypeStr=boolean
  O2 : Inport  Port=8  OutDataTypeStr=boolean
  O3 : Inport  Port=9  OutDataTypeStr=boolean
  LD : Inport  Port=10  OutDataTypeStr=boolean
  Cyber : Subsystem
  M : Memory
  M1 : Memory
  M2 : Memory
  Physical : Subsystem
  S1 : Subsystem
  S2 : Subsystem
  S3 : Subsystem
  W1Pos : Outport
  W2Pos : Outport  Port=2
  W3Pos : Outport  Port=3
  wires:
  DW2/1 -> Cyber/5(DW2)
  S2/1(SensorOut) -> M1/1
  Physical/2(W2) -> S2/1(PhyMeasure), W2Pos/1
  DW1/1 -> Cyber/4(DW1)
  M/1 -> Cyber/1(PosW1)
  Physical/3(W3) -> S3/1(PhyMeasure), W3Pos/1
  M1/1 -> Cyber/2(PosW2)
  DW3/1 -> Cyber/6(DW3)
  P1W3/1 -> Cyber/9(P1W3)
  O3/1 -> Cyber/12(OW3)
  P1W2/1 -> Cyber/7(P1W2)
  M2/1 -> Cyber/3(PosW3)
  Cyber/2(W2) -> Physical/2(InW2)
  Cyber/1(W1) -> Physical/1(InW1)
  O1/1 -> Cyber/10(OW1)
  LD/1 -> Cyber/13(LD)
  Cyber/3(W3) -> Physical/3(InW3)
  O2/1 -> Cyber/11(OW2)
  S3/1(SensorOut) -> M2/1
  Physical/1(W1) -> S1/1(PhyMeasure), W1Pos/1
  S1/1(SensorOut) -> M/1
  P2W3/1 -> Cyber/8(P2W3)

== system c00010M_harness/M025 ==
  DW1 : Inport  OutMin=0  OutMax=4  OutDataTypeStr=int8
  DW2 : Inport  Port=2  OutMin=0  OutMax=4  OutDataTypeStr=int8
  DW3 : Inport  Port=3  OutMin=0  OutMax=4  OutDataTypeStr=int8
  P1W2 : Inport  Port=4  OutMin=0  OutMax=4  OutDataTypeStr=int8
  P2W3 : Inport  Port=5  OutMin=0  OutMax=4  OutDataTypeStr=int8
  P1W3 : Inport  Port=6  OutMin=0  OutMax=4  OutDataTypeStr=int8
  O1 : Inport  Port=7  OutDataTypeStr=boolean
  O2 : Inport  Port=8  OutDataTypeStr=boolean
  O3 : Inport  Port=9  OutDataTypeStr=boolean
  LD : Inport  Port=10  OutDataTypeStr=boolean
  Cyber : Subsystem
  M : Memory
  M1 : Memory
  M2 : Memory
  Physical : Subsystem
  S1 : Subsystem
  S2 : Subsystem
  S3 : Subsystem
  W1Pos : Outport
  W2Pos : Outport  Port=2
  W3Pos : Outport  Port=3
  wires:
  DW2/1 -> Cyber/5(DW2)
  S2/1(SensorOut) -> M1/1
  Physical/2(W2) -> S2/1(PhyMeasure), W2Pos/1
  DW1/1 -> Cyber/4(DW1)
  M/1 -> Cyber/1(PosW1)
  Physical/3(W3) -> S3/1(PhyMeasure), W3Pos/1
  M1/1 -> Cyber/2(PosW2)
  DW3/1 -> Cyber/6(DW3)
  P1W3/1 -> Cyber/9(P1W3)
  O3/1 -> Cyber/12(OW3)
  P1W2/1 -> Cyber/7(P1W2)
  M2/1 -> Cyber/3(PosW3)
  Cyber/2(W2) -> Physical/2(InW2)
  Cyber/1(W1) -> Physical/1(InW1)
  O1/1 -> Cyber/10(OW1)
  LD/1 -> Cyber/13(LD)
  Cyber/3(W3) -> Physical/3(InW3)
  O2/1 -> Cyber/11(OW2)
  S3/1(SensorOut) -> M2/1
  Physical/1(W1) -> S1/1(PhyMeasure), W1Pos/1
  S1/1(SensorOut) -> M/1
  P2W3/1 -> Cyber/8(P2W3)

== system c00010M_harness/M030 ==
  DW1 : Inport  OutMin=0  OutMax=4  OutDataTypeStr=int8
  DW2 : Inport  Port=2  OutMin=0  OutMax=4  OutDataTypeStr=int8
  DW3 : Inport  Port=3  OutMin=0  OutMax=4  OutDataTypeStr=int8
  P1W2 : Inport  Port=4  OutMin=0  OutMax=4  OutDataTypeStr=int8
  P2W3 : Inport  Port=5  OutMin=0  OutMax=4  OutDataTypeStr=int8
  P1W3 : Inport  Port=6  OutMin=0  OutMax=4  OutDataTypeStr=int8
  O1 : Inport  Port=7  OutDataTypeStr=boolean
  O2 : Inport  Port=8  OutDataTypeStr=boolean
  O3 : Inport  Port=9  OutDataTypeStr=boolean
  LD : Inport  Port=10  OutDataTypeStr=boolean
  Cyber : Subsystem
  M : Memory
  M1 : Memory
  M2 : Memory
  Physical : Subsystem
  S1 : Subsystem
  S2 : Subsystem
  S3 : Subsystem
  W1Pos : Outport
  W2Pos : Outport  Port=2
  W3Pos : Outport  Port=3
  wires:
  DW2/1 -> Cyber/5(DW2)
  S2/1(SensorOut) -> M1/1
  Physical/2(W2) -> S2/1(PhyMeasure), W2Pos/1
  DW1/1 -> Cyber/4(DW1)
  M/1 -> Cyber/1(PosW1)
  Physical/3(W3) -> S3/1(PhyMeasure), W3Pos/1
  M1/1 -> Cyber/2(PosW2)
  DW3/1 -> Cyber/6(DW3)
  P1W3/1 -> Cyber/9(P1W3)
  O3/1 -> Cyber/12(OW3)
  P1W2/1 -> Cyber/7(P1W2)
  M2/1 -> Cyber/3(PosW3)
  Cyber/2(W2) -> Physical/2(InW2)
  Cyber/1(W1) -> Physical/1(InW1)
  O1/1 -> Cyber/10(OW1)
  LD/1 -> Cyber/13(LD)
  Cyber/3(W3) -> Physical/3(InW3)
  O2/1 -> Cyber/11(OW2)
  S3/1(SensorOut) -> M2/1
  Physical/1(W1) -> S1/1(PhyMeasure), W1Pos/1
  S1/1(SensorOut) -> M/1
  P2W3/1 -> Cyber/8(P2W3)

== system c00010M_harness/M037 ==
  DW1 : Inport  OutMin=0  OutMax=4  OutDataTypeStr=int8
  DW2 : Inport  Port=2  OutMin=0  OutMax=4  OutDataTypeStr=int8
  DW3 : Inport  Port=3  OutMin=0  OutMax=4  OutDataTypeStr=int8
  P1W2 : Inport  Port=4  OutMin=0  OutMax=4  OutDataTypeStr=int8
  P2W3 : Inport  Port=5  OutMin=0  OutMax=4  OutDataTypeStr=int8
  P1W3 : Inport  Port=6  OutMin=0  OutMax=4  OutDataTypeStr=int8
  O1 : Inport  Port=7  OutDataTypeStr=boolean
  O2 : Inport  Port=8  OutDataTypeStr=boolean
  O3 : Inport  Port=9  OutDataTypeStr=boolean
  LD : Inport  Port=10  OutDataTypeStr=boolean
  Cyber : Subsystem
  M : Memory
  M1 : Memory
  M2 : Memory
  Physical : Subsystem
  S1 : Subsystem
  S2 : Subsystem
  S3 : Subsystem
  W1Pos : Outport
  W2Pos : Outport  Port=2
  W3Pos : Outport  Port=3
  wires:
  DW2/1 -> Cyber/5(DW2)
  S2/1(SensorOut) -> M1/1
  Physical/2(W2) -> S2/1(PhyMeasure), W2Pos/1
  DW1/1 -> Cyber/4(DW1)
  M/1 -> Cyber/1(PosW1)
  Physical/3(W3) -> S3/1(PhyMeasure), W3Pos/1
  M1/1 -> Cyber/2(PosW2)
  DW3/1 -> Cyber/6(DW3)
  P1W3/1 -> Cyber/9(P1W3)
  O3/1 -> Cyber/12(OW3)
  P1W2/1 -> Cyber/7(P1W2)
  M2/1 -> Cyber/3(PosW3)
  Cyber/2(W2) -> Physical/2(InW2)
  Cyber/1(W1) -> Physical/1(InW1)
  O1/1 -> Cyber/10(OW1)
  LD/1 -> Cyber/13(LD)
  Cyber/3(W3) -> Physical/3(InW3)
  O2/1 -> Cyber/11(OW2)
  S3/1(SensorOut) -> M2/1
  Physical/1(W1) -> S1/1(PhyMeasure), W1Pos/1
  S1/1(SensorOut) -> M/1
  P2W3/1 -> Cyber/8(P2W3)

== system c00010M_harness/M040 ==
  DW1 : Inport  OutMin=0  OutMax=4  OutDataTypeStr=int8
  DW2 : Inport  Port=2  OutMin=0  OutMax=4  OutDataTypeStr=int8
  DW3 : Inport  Port=3  OutMin=0  OutMax=4  OutDataTypeStr=int8
  P1W2 : Inport  Port=4  OutMin=0  OutMax=4  OutDataTypeStr=int8
  P2W3 : Inport  Port=5  OutMin=0  OutMax=4  OutDataTypeStr=int8
  P1W3 : Inport  Port=6  OutMin=0  OutMax=4  OutDataTypeStr=int8
  O1 : Inport  Port=7  OutDataTypeStr=boolean
  O2 : Inport  Port=8  OutDataTypeStr=boolean
  O3 : Inport  Port=9  OutDataTypeStr=boolean
  LD : Inport  Port=10  OutDataTypeStr=boolean
  Cyber : Subsystem
  M : Memory
  M1 : Memory
  M2 : Memory
  Physical : Subsystem
  S1 : Subsystem
  S2 : Subsystem
  S3 : Subsystem
  W1Pos : Outport
  W2Pos : Outport  Port=2
  W3Pos : Outport  Port=3
  wires:
  DW2/1 -> Cyber/5(DW2)
  S2/1(SensorOut) -> M1/1
  Physical/2(W2) -> S2/1(PhyMeasure), W2Pos/1
  DW1/1 -> Cyber/4(DW1)
  M/1 -> Cyber/1(PosW1)
  Physical/3(W3) -> S3/1(PhyMeasure), W3Pos/1
  M1/1 -> Cyber/2(PosW2)
  DW3/1 -> Cyber/6(DW3)
  P1W3/1 -> Cyber/9(P1W3)
  O3/1 -> Cyber/12(OW3)
  P1W2/1 -> Cyber/7(P1W2)
  M2/1 -> Cyber/3(PosW3)
  Cyber/2(W2) -> Physical/2(InW2)
  Cyber/1(W1) -> Physical/1(InW1)
  O1/1 -> Cyber/10(OW1)
  LD/1 -> Cyber/13(LD)
  Cyber/3(W3) -> Physical/3(InW3)
  O2/1 -> Cyber/11(OW2)
  S3/1(SensorOut) -> M2/1
  Physical/1(W1) -> S1/1(PhyMeasure), W1Pos/1
  S1/1(SensorOut) -> M/1
  P2W3/1 -> Cyber/8(P2W3)

== system c00010M_harness/M054 ==
  DW1 : Inport  OutMin=0  OutMax=4  OutDataTypeStr=int8
  DW2 : Inport  Port=2  OutMin=0  OutMax=4  OutDataTypeStr=int8
  DW3 : Inport  Port=3  OutMin=0  OutMax=4  OutDataTypeStr=int8
  P1W2 : Inport  Port=4  OutMin=0  OutMax=4  OutDataTypeStr=int8
  P2W3 : Inport  Port=5  OutMin=0  OutMax=4  OutDataTypeStr=int8
  P1W3 : Inport  Port=6  OutMin=0  OutMax=4  OutDataTypeStr=int8
  O1 : Inport  Port=7  OutDataTypeStr=boolean
  O2 : Inport  Port=8  OutDataTypeStr=boolean
  O3 : Inport  Port=9  OutDataTypeStr=boolean
  LD : Inport  Port=10  OutDataTypeStr=boolean
  Cyber : Subsystem
  M : Memory
  M1 : Memory
  M2 : Memory
  Physical : Subsystem
  S1 : Subsystem
  S2 : Subsystem
  S3 : Subsystem
  W1Pos : Outport
  W2Pos : Outport  Port=2
  W3Pos : Outport  Port=3
  wires:
  DW2/1 -> Cyber/5(DW2)
  S2/1(SensorOut) -> M1/1
  Physical/2(W2) -> S2/1(PhyMeasure), W2Pos/1
  DW1/1 -> Cyber/4(DW1)
  M/1 -> Cyber/1(PosW1)
  Physical/3(W3) -> S3/1(PhyMeasure), W3Pos/1
  M1/1 -> Cyber/2(PosW2)
  DW3/1 -> Cyber/6(DW3)
  P1W3/1 -> Cyber/9(P1W3)
  O3/1 -> Cyber/12(OW3)
  P1W2/1 -> Cyber/7(P1W2)
  M2/1 -> Cyber/3(PosW3)
  Cyber/2(W2) -> Physical/2(InW2)
  Cyber/1(W1) -> Physical/1(InW1)
  O1/1 -> Cyber/10(OW1)
  LD/1 -> Cyber/13(LD)
  Cyber/3(W3) -> Physical/3(InW3)
  O2/1 -> Cyber/11(OW2)
  S3/1(SensorOut) -> M2/1
  Physical/1(W1) -> S1/1(PhyMeasure), W1Pos/1
  S1/1(SensorOut) -> M/1
  P2W3/1 -> Cyber/8(P2W3)

== system c00010M_harness/CPSUT/Cyber ==
  note: D = Driver (W1)
      | P1 = Passenger 1 (W2)
      | P2 = Passenger 2 (W3)
      | P3 = Passenger 3 (W4)
      | O = Obstacle
      | C = Control
      | Pri = Prioritizer
      | LD = LockDriver
      | PosW = PositionWindow
      | WL = WindowLogic
      | OW = ObstacleWindow
      | CWXC = ControlWindowXCentralized
      | S = Sensor
      | L = Lock
      | WPos = WindowPosition
      | M = Memory
      | InW = InputWindow
      | WIn = WindowInput
  note: 1: SUBE
      | 0: PARADO
      | -1 BAJA
  note: USERS
      | ---------------------------------
      | 0: None
      | 1: Ventana Arriba
      | 2: Ventana hasta arriba
      | 3: Ventana abajo
      | 4: Ventana hasta abajo
  note: Sensors
  note: Users
  note: Sensors
  note: Users
  note: Sensors
  note: Users
  note: Users
  note: Inputs for window 4
  note: Inputs for window 3
  note: Inputs for Window 2
  note: Inputs For Window1
  note: Sensors
  PosW1 : Inport
  PosW2 : Inport  Port=2
  PosW3 : Inport  Port=3
  DW1 : Inport  Port=4
  DW2 : Inport  Port=5
  DW3 : Inport  Port=6
  P1W2 : Inport  Port=7
  P2W3 : Inport  Port=8
  P1W3 : Inport  Port=9
  OW1 : Inport  Port=10
  OW2 : Inport  Port=11
  OW3 : Inport  Port=12
  LD : Inport  Port=13
  Pri : Subsystem
  Pri1 : Subsystem
  WL : Subsystem
  WL1 : Subsystem
  WL2 : Subsystem
  W1 : Outport
  W2 : Outport  Port=2
  W3 : Outport  Port=3
  wires:
  LD/1 -> WL2/4(L)
  PosW1/1 -> WL/1(WPos)
  OW1/1 -> WL/3(OW)
  WL/1(WindowLogicOutput) -> W1/1
  Pri/1(User) -> WL1/2(User)
  DW2/1 -> Pri/1(D)
  P1W2/1 -> Pri/2(P)
  PosW2/1 -> WL1/1(WPos)
  OW2/1 -> WL1/3(OW)
  WL1/1(WindowLogicOutput) -> W2/1
  Pri1/1(User) -> WL2/2(User)
  PosW3/1 -> WL2/1(WPos)
  OW3/1 -> WL2/3(OW)
  DW3/1 -> Pri1/1(D)
  P2W3/1 -> Pri1/2(P)
  P1W3/1 -> Pri1/3(P1)
  WL2/1(WindowLogicOutput) -> W3/1
  DW1/1 -> WL/2(User)

== system c00010M_harness/CPSUT/Physical ==
  InW1 : Inport
  InW2 : Inport  Port=2
  InW3 : Inport  Port=3
  W : Subsystem
  W5 : Subsystem
  W6 : Subsystem
  W1 : Outport
  W2 : Outport  Port=2
  W3 : Outport  Port=3
  wires:
  InW1/1 -> W/1(WIn)
  InW2/1 -> W5/1(WIn)
  InW3/1 -> W6/1(WIn)
  W/1(WPos) -> W1/1
  W5/1(WPos) -> W2/1
  W6/1(WPos) -> W3/1

== system c00010M_harness/CPSUT/S1 ==
  PhyMeasure : Inport
  SensorOut : Outport
  wires:
  PhyMeasure/1 -> SensorOut/1

== system c00010M_harness/CPSUT/S2 ==
  PhyMeasure : Inport
  SensorOut : Outport
  wires:
  PhyMeasure/1 -> SensorOut/1

== system c00010M_harness/CPSUT/S3 ==
  PhyMeasure : Inport
  SensorOut : Outport
  wires:
  PhyMeasure/1 -> SensorOut/1

== system c00010M_harness/M001/Cyber ==
  note: D = Driver (W1)
      | P1 = Passenger 1 (W2)
      | P2 = Passenger 2 (W3)
      | P3 = Passenger 3 (W4)
      | O = Obstacle
      | C = Control
      | Pri = Prioritizer
      | LD = LockDriver
      | PosW = PositionWindow
      | WL = WindowLogic
      | OW = ObstacleWindow
      | CWXC = ControlWindowXCentralized
      | S = Sensor
      | L = Lock
      | WPos = WindowPosition
      | M = Memory
      | InW = InputWindow
      | WIn = WindowInput
  note: 1: SUBE
      | 0: PARADO
      | -1 BAJA
  note: USERS
      | ---------------------------------
      | 0: None
      | 1: Ventana Arriba
      | 2: Ventana hasta arriba
      | 3: Ventana abajo
      | 4: Ventana hasta abajo
  note: Sensors
  note: Users
  note: Sensors
  note: Users
  note: Sensors
  note: Users
  note: Users
  note: Inputs for window 4
  note: Inputs for window 3
  note: Inputs for Window 2
  note: Inputs For Window1
  note: Sensors
  PosW1 : Inport
  PosW2 : Inport  Port=2
  PosW3 : Inport  Port=3
  DW1 : Inport  Port=4
  DW2 : Inport  Port=5
  DW3 : Inport  Port=6
  P1W2 : Inport  Port=7
  P2W3 : Inport  Port=8
  P1W3 : Inport  Port=9
  OW1 : Inport  Port=10
  OW2 : Inport  Port=11
  OW3 : Inport  Port=12
  LD : Inport  Port=13
  Pri : Subsystem
  Pri1 : Subsystem
  WL : Subsystem
  WL1 : Subsystem
  WL2 : Subsystem
  W1 : Outport
  W2 : Outport  Port=2
  W3 : Outport  Port=3
  wires:
  LD/1 -> WL2/4(L)
  PosW1/1 -> WL/1(WPos)
  OW1/1 -> WL/3(OW)
  WL/1(WindowLogicOutput) -> W1/1
  Pri/1(User) -> WL1/2(User)
  DW2/1 -> Pri/1(D)
  P1W2/1 -> Pri/2(P)
  PosW2/1 -> WL1/1(WPos)
  OW2/1 -> WL1/3(OW)
  WL1/1(WindowLogicOutput) -> W2/1
  Pri1/1(User) -> WL2/2(User)
  PosW3/1 -> WL2/1(WPos)
  OW3/1 -> WL2/3(OW)
  DW3/1 -> Pri1/1(D)
  P2W3/1 -> Pri1/2(P)
  P1W3/1 -> Pri1/3(P1)
  WL2/1(WindowLogicOutput) -> W3/1
  DW1/1 -> WL/2(User)

== system c00010M_harness/M001/Physical ==
  InW1 : Inport
  InW2 : Inport  Port=2
  InW3 : Inport  Port=3
  W : Subsystem
  W5 : Subsystem
  W6 : Subsystem
  W1 : Outport
  W2 : Outport  Port=2
  W3 : Outport  Port=3
  wires:
  InW1/1 -> W/1(WIn)
  InW2/1 -> W5/1(WIn)
  InW3/1 -> W6/1(WIn)
  W/1(WPos) -> W1/1
  W5/1(WPos) -> W2/1
  W6/1(WPos) -> W3/1

== system c00010M_harness/M001/S1 ==
  PhyMeasure : Inport
  SensorOut : Outport
  wires:
  PhyMeasure/1 -> SensorOut/1

== system c00010M_harness/M001/S2 ==
  PhyMeasure : Inport
  SensorOut : Outport
  wires:
  PhyMeasure/1 -> SensorOut/1

== system c00010M_harness/M001/S3 ==
  PhyMeasure : Inport
  SensorOut : Outport
  wires:
  PhyMeasure/1 -> SensorOut/1

== system c00010M_harness/M008/Cyber ==
  note: Sensors
  note: Inputs For Window1
  note: Inputs for Window 2
  note: Inputs for window 3
  note: Inputs for window 4
  note: Users
  note: Users
  note: Sensors
  note: Users
  note: Sensors
  note: Users
  note: Sensors
  note: USERS
      | ---------------------------------
      | 0: None
      | 1: Ventana Arriba
      | 2: Ventana hasta arriba
      | 3: Ventana abajo
      | 4: Ventana hasta abajo
  note: 1: SUBE
      | 0: PARADO
      | -1 BAJA
  note: D = Driver (W1)
      | P1 = Passenger 1 (W2)
      | P2 = Passenger 2 (W3)
      | P3 = Passenger 3 (W4)
      | O = Obstacle
      | C = Control
      | Pri = Prioritizer
      | LD = LockDriver
      | PosW = PositionWindow
      | WL = WindowLogic
      | OW = ObstacleWindow
      | CWXC = ControlWindowXCentralized
      | S = Sensor
      | L = Lock
      | WPos = WindowPosition
      | M = Memory
      | InW = InputWindow
      | WIn = WindowInput
  PosW1 : Inport
  PosW2 : Inport  Port=2
  PosW3 : Inport  Port=3
  DW1 : Inport  Port=4
  DW2 : Inport  Port=5
  DW3 : Inport  Port=6
  P1W2 : Inport  Port=7
  P2W3 : Inport  Port=8
  P1W3 : Inport  Port=9
  OW1 : Inport  Port=10
  OW2 : Inport  Port=11
  OW3 : Inport  Port=12
  LD : Inport  Port=13
  Pri : Subsystem
  Pri1 : Subsystem
  WL : Subsystem
  WL1 : Subsystem
  WL2 : Subsystem
  W1 : Outport
  W2 : Outport  Port=2
  W3 : Outport  Port=3
  wires:
  WL2/1(WindowLogicOutput) -> W3/1
  P1W3/1 -> Pri1/3(P1)
  P2W3/1 -> Pri1/2(P)
  DW3/1 -> Pri1/1(D)
  OW3/1 -> WL2/3(OW)
  PosW3/1 -> WL2/1(WPos)
  Pri1/1(User) -> WL2/2(User)
  WL1/1(WindowLogicOutput) -> W2/1
  OW2/1 -> WL1/3(OW)
  PosW2/1 -> WL1/1(WPos)
  P1W2/1 -> Pri/2(P)
  DW2/1 -> Pri/1(D)
  Pri/1(User) -> WL1/2(User)
  WL/1(WindowLogicOutput) -> W1/1
  OW1/1 -> WL/3(OW)
  PosW1/1 -> WL/1(WPos)
  LD/1 -> WL2/4(L)
  DW1/1 -> WL/2(User)

== system c00010M_harness/M008/Physical ==
  InW1 : Inport
  InW2 : Inport  Port=2
  InW3 : Inport  Port=3
  W : Subsystem
  W5 : Subsystem
  W6 : Subsystem
  W1 : Outport
  W2 : Outport  Port=2
  W3 : Outport  Port=3
  wires:
  W6/1(WPos) -> W3/1
  W5/1(WPos) -> W2/1
  W/1(WPos) -> W1/1
  InW3/1 -> W6/1(WIn)
  InW2/1 -> W5/1(WIn)
  InW1/1 -> W/1(WIn)

== system c00010M_harness/M008/S1 ==
  PhyMeasure : Inport
  SensorOut : Outport
  wires:
  PhyMeasure/1 -> SensorOut/1

== system c00010M_harness/M008/S2 ==
  PhyMeasure : Inport
  SensorOut : Outport
  wires:
  PhyMeasure/1 -> SensorOut/1

== system c00010M_harness/M008/S3 ==
  PhyMeasure : Inport
  SensorOut : Outport
  wires:
  PhyMeasure/1 -> SensorOut/1

== system c00010M_harness/M011/Cyber ==
  note: Sensors
  note: Inputs For Window1
  note: Inputs for Window 2
  note: Inputs for window 3
  note: Inputs for window 4
  note: Users
  note: Users
  note: Sensors
  note: Users
  note: Sensors
  note: Users
  note: Sensors
  note: USERS
      | ---------------------------------
      | 0: None
      | 1: Ventana Arriba
      | 2: Ventana hasta arriba
      | 3: Ventana abajo
      | 4: Ventana hasta abajo
  note: 1: SUBE
      | 0: PARADO
      | -1 BAJA
  note: D = Driver (W1)
      | P1 = Passenger 1 (W2)
      | P2 = Passenger 2 (W3)
      | P3 = Passenger 3 (W4)
      | O = Obstacle
      | C = Control
      | Pri = Prioritizer
      | LD = LockDriver
      | PosW = PositionWindow
      | WL = WindowLogic
      | OW = ObstacleWindow
      | CWXC = ControlWindowXCentralized
      | S = Sensor
      | L = Lock
      | WPos = WindowPosition
      | M = Memory
      | InW = InputWindow
      | WIn = WindowInput
  PosW1 : Inport
  PosW2 : Inport  Port=2
  PosW3 : Inport  Port=3
  DW1 : Inport  Port=4
  DW2 : Inport  Port=5
  DW3 : Inport  Port=6
  P1W2 : Inport  Port=7
  P2W3 : Inport  Port=8
  P1W3 : Inport  Port=9
  OW1 : Inport  Port=10
  OW2 : Inport  Port=11
  OW3 : Inport  Port=12
  LD : Inport  Port=13
  Pri : Subsystem
  Pri1 : Subsystem
  WL : Subsystem
  WL1 : Subsystem
  WL2 : Subsystem
  W1 : Outport
  W2 : Outport  Port=2
  W3 : Outport  Port=3
  wires:
  WL2/1(WindowLogicOutput) -> W3/1
  P1W3/1 -> Pri1/3(P1)
  P2W3/1 -> Pri1/2(P)
  DW3/1 -> Pri1/1(D)
  OW3/1 -> WL2/3(OW)
  PosW3/1 -> WL2/1(WPos)
  Pri1/1(User) -> WL2/2(User)
  WL1/1(WindowLogicOutput) -> W2/1
  OW2/1 -> WL1/3(OW)
  PosW2/1 -> WL1/1(WPos)
  P1W2/1 -> Pri/2(P)
  DW2/1 -> Pri/1(D)
  Pri/1(User) -> WL1/2(User)
  WL/1(WindowLogicOutput) -> W1/1
  OW1/1 -> WL/3(OW)
  PosW1/1 -> WL/1(WPos)
  LD/1 -> WL2/4(L)
  DW1/1 -> WL/2(User)

== system c00010M_harness/M011/Physical ==
  InW1 : Inport
  InW2 : Inport  Port=2
  InW3 : Inport  Port=3
  W : Subsystem
  W5 : Subsystem
  W6 : Subsystem
  W1 : Outport
  W2 : Outport  Port=2
  W3 : Outport  Port=3
  wires:
  W6/1(WPos) -> W3/1
  W5/1(WPos) -> W2/1
  W/1(WPos) -> W1/1
  InW3/1 -> W6/1(WIn)
  InW2/1 -> W5/1(WIn)
  InW1/1 -> W/1(WIn)

== system c00010M_harness/M011/S1 ==
  PhyMeasure : Inport
  SensorOut : Outport
  wires:
  PhyMeasure/1 -> SensorOut/1

== system c00010M_harness/M011/S2 ==
  PhyMeasure : Inport
  SensorOut : Outport
  wires:
  PhyMeasure/1 -> SensorOut/1

== system c00010M_harness/M011/S3 ==
  PhyMeasure : Inport
  SensorOut : Outport
  wires:
  PhyMeasure/1 -> SensorOut/1

== system c00010M_harness/M025/Cyber ==
  note: Sensors
  note: Inputs For Window1
  note: Inputs for Window 2
  note: Inputs for window 3
  note: Inputs for window 4
  note: Users
  note: Users
  note: Sensors
  note: Users
  note: Sensors
  note: Users
  note: Sensors
  note: USERS
      | ---------------------------------
      | 0: None
      | 1: Ventana Arriba
      | 2: Ventana hasta arriba
      | 3: Ventana abajo
      | 4: Ventana hasta abajo
  note: 1: SUBE
      | 0: PARADO
      | -1 BAJA
  note: D = Driver (W1)
      | P1 = Passenger 1 (W2)
      | P2 = Passenger 2 (W3)
      | P3 = Passenger 3 (W4)
      | O = Obstacle
      | C = Control
      | Pri = Prioritizer
      | LD = LockDriver
      | PosW = PositionWindow
      | WL = WindowLogic
      | OW = ObstacleWindow
      | CWXC = ControlWindowXCentralized
      | S = Sensor
      | L = Lock
      | WPos = WindowPosition
      | M = Memory
      | InW = InputWindow
      | WIn = WindowInput
  PosW1 : Inport
  PosW2 : Inport  Port=2
  PosW3 : Inport  Port=3
  DW1 : Inport  Port=4
  DW2 : Inport  Port=5
  DW3 : Inport  Port=6
  P1W2 : Inport  Port=7
  P2W3 : Inport  Port=8
  P1W3 : Inport  Port=9
  OW1 : Inport  Port=10
  OW2 : Inport  Port=11
  OW3 : Inport  Port=12
  LD : Inport  Port=13
  Pri : Subsystem
  Pri1 : Subsystem
  WL : Subsystem
  WL1 : Subsystem
  WL2 : Subsystem
  W1 : Outport
  W2 : Outport  Port=2
  W3 : Outport  Port=3
  wires:
  WL2/1(WindowLogicOutput) -> W3/1
  P1W3/1 -> Pri1/3(P1)
  P2W3/1 -> Pri1/2(P)
  DW3/1 -> Pri1/1(D)
  OW3/1 -> WL2/3(OW)
  PosW3/1 -> WL2/1(WPos)
  Pri1/1(User) -> WL2/2(User)
  WL1/1(WindowLogicOutput) -> W2/1
  OW2/1 -> WL1/3(OW)
  PosW2/1 -> WL1/1(WPos)
  P1W2/1 -> Pri/2(P)
  DW2/1 -> Pri/1(D)
  Pri/1(User) -> WL1/2(User)
  WL/1(WindowLogicOutput) -> W1/1
  OW1/1 -> WL/3(OW)
  PosW1/1 -> WL/1(WPos)
  LD/1 -> WL2/4(L)
  DW1/1 -> WL/2(User)

== system c00010M_harness/M025/Physical ==
  InW1 : Inport
  InW2 : Inport  Port=2
  InW3 : Inport  Port=3
  W : Subsystem
  W5 : Subsystem
  W6 : Subsystem
  W1 : Outport
  W2 : Outport  Port=2
  W3 : Outport  Port=3
  wires:
  W6/1(WPos) -> W3/1
  W5/1(WPos) -> W2/1
  W/1(WPos) -> W1/1
  InW3/1 -> W6/1(WIn)
  InW2/1 -> W5/1(WIn)
  InW1/1 -> W/1(WIn)

== system c00010M_harness/M025/S1 ==
  PhyMeasure : Inport
  SensorOut : Outport
  wires:
  PhyMeasure/1 -> SensorOut/1

== system c00010M_harness/M025/S2 ==
  PhyMeasure : Inport
  SensorOut : Outport
  wires:
  PhyMeasure/1 -> SensorOut/1

== system c00010M_harness/M025/S3 ==
  PhyMeasure : Inport
  SensorOut : Outport
  wires:
  PhyMeasure/1 -> SensorOut/1

== system c00010M_harness/M030/Cyber ==
  note: Sensors
  note: Inputs For Window1
  note: Inputs for Window 2
  note: Inputs for window 3
  note: Inputs for window 4
  note: Users
  note: Users
  note: Sensors
  note: Users
  note: Sensors
  note: Users
  note: Sensors
  note: USERS
      | ---------------------------------
      | 0: None
      | 1: Ventana Arriba
      | 2: Ventana hasta arriba
      | 3: Ventana abajo
      | 4: Ventana hasta abajo
  note: 1: SUBE
      | 0: PARADO
      | -1 BAJA
  note: D = Driver (W1)
      | P1 = Passenger 1 (W2)
      | P2 = Passenger 2 (W3)
      | P3 = Passenger 3 (W4)
      | O = Obstacle
      | C = Control
      | Pri = Prioritizer
      | LD = LockDriver
      | PosW = PositionWindow
      | WL = WindowLogic
      | OW = ObstacleWindow
      | CWXC = ControlWindowXCentralized
      | S = Sensor
      | L = Lock
      | WPos = WindowPosition
      | M = Memory
      | InW = InputWindow
      | WIn = WindowInput
  PosW1 : Inport
  PosW2 : Inport  Port=2
  PosW3 : Inport  Port=3
  DW1 : Inport  Port=4
  DW2 : Inport  Port=5
  DW3 : Inport  Port=6
  P1W2 : Inport  Port=7
  P2W3 : Inport  Port=8
  P1W3 : Inport  Port=9
  OW1 : Inport  Port=10
  OW2 : Inport  Port=11
  OW3 : Inport  Port=12
  LD : Inport  Port=13
  Pri : Subsystem
  Pri1 : Subsystem
  WL : Subsystem
  WL1 : Subsystem
  WL2 : Subsystem
  W1 : Outport
  W2 : Outport  Port=2
  W3 : Outport  Port=3
  wires:
  WL2/1(WindowLogicOutput) -> W3/1
  P1W3/1 -> Pri1/3(P1)
  P2W3/1 -> Pri1/2(P)
  DW3/1 -> Pri1/1(D)
  OW3/1 -> WL2/3(OW)
  PosW3/1 -> WL2/1(WPos)
  Pri1/1(User) -> WL2/2(User)
  WL1/1(WindowLogicOutput) -> W2/1
  OW2/1 -> WL1/3(OW)
  PosW2/1 -> WL1/1(WPos)
  P1W2/1 -> Pri/2(P)
  DW2/1 -> Pri/1(D)
  Pri/1(User) -> WL1/2(User)
  WL/1(WindowLogicOutput) -> W1/1
  OW1/1 -> WL/3(OW)
  PosW1/1 -> WL/1(WPos)
  LD/1 -> WL2/4(L)
  DW1/1 -> WL/2(User)

== system c00010M_harness/M030/Physical ==
  InW1 : Inport
  InW2 : Inport  Port=2
  InW3 : Inport  Port=3
  W : Subsystem
  W5 : Subsystem
  W6 : Subsystem
  W1 : Outport
  W2 : Outport  Port=2
  W3 : Outport  Port=3
  wires:
  W6/1(WPos) -> W3/1
  W5/1(WPos) -> W2/1
  W/1(WPos) -> W1/1
  InW3/1 -> W6/1(WIn)
  InW2/1 -> W5/1(WIn)
  InW1/1 -> W/1(WIn)

== system c00010M_harness/M030/S1 ==
  PhyMeasure : Inport
  SensorOut : Outport
  wires:
  PhyMeasure/1 -> SensorOut/1

== system c00010M_harness/M030/S2 ==
  PhyMeasure : Inport
  SensorOut : Outport
  wires:
  PhyMeasure/1 -> SensorOut/1

== system c00010M_harness/M030/S3 ==
  PhyMeasure : Inport
  SensorOut : Outport
  wires:
  PhyMeasure/1 -> SensorOut/1

== system c00010M_harness/M037/Cyber ==
  note: Sensors
  note: Inputs For Window1
  note: Inputs for Window 2
  note: Inputs for window 3
  note: Inputs for window 4
  note: Users
  note: Users
  note: Sensors
  note: Users
  note: Sensors
  note: Users
  note: Sensors
  note: USERS
      | ---------------------------------
      | 0: None
      | 1: Ventana Arriba
      | 2: Ventana hasta arriba
      | 3: Ventana abajo
      | 4: Ventana hasta abajo
  note: 1: SUBE
      | 0: PARADO
      | -1 BAJA
  note: D = Driver (W1)
      | P1 = Passenger 1 (W2)
      | P2 = Passenger 2 (W3)
      | P3 = Passenger 3 (W4)
      | O = Obstacle
      | C = Control
      | Pri = Prioritizer
      | LD = LockDriver
      | PosW = PositionWindow
      | WL = WindowLogic
      | OW = ObstacleWindow
      | CWXC = ControlWindowXCentralized
      | S = Sensor
      | L = Lock
      | WPos = WindowPosition
      | M = Memory
      | InW = InputWindow
      | WIn = WindowInput
  PosW1 : Inport
  PosW2 : Inport  Port=2
  PosW3 : Inport  Port=3
  DW1 : Inport  Port=4
  DW2 : Inport  Port=5
  DW3 : Inport  Port=6
  P1W2 : Inport  Port=7
  P2W3 : Inport  Port=8
  P1W3 : Inport  Port=9
  OW1 : Inport  Port=10
  OW2 : Inport  Port=11
  OW3 : Inport  Port=12
  LD : Inport  Port=13
  Pri : Subsystem
  Pri1 : Subsystem
  WL : Subsystem
  WL1 : Subsystem
  WL2 : Subsystem
  W1 : Outport
  W2 : Outport  Port=2
  W3 : Outport  Port=3
  wires:
  WL2/1(WindowLogicOutput) -> W3/1
  P1W3/1 -> Pri1/3(P1)
  P2W3/1 -> Pri1/2(P)
  DW3/1 -> Pri1/1(D)
  OW3/1 -> WL2/3(OW)
  PosW3/1 -> WL2/1(WPos)
  Pri1/1(User) -> WL2/2(User)
  WL1/1(WindowLogicOutput) -> W2/1
  OW2/1 -> WL1/3(OW)
  PosW2/1 -> WL1/1(WPos)
  P1W2/1 -> Pri/2(P)
  DW2/1 -> Pri/1(D)
  Pri/1(User) -> WL1/2(User)
  WL/1(WindowLogicOutput) -> W1/1
  OW1/1 -> WL/3(OW)
  PosW1/1 -> WL/1(WPos)
  LD/1 -> WL2/4(L)
  DW1/1 -> WL/2(User)

== system c00010M_harness/M037/Physical ==
  InW1 : Inport
  InW2 : Inport  Port=2
  InW3 : Inport  Port=3
  W : Subsystem
  W5 : Subsystem
  W6 : Subsystem
  W1 : Outport
  W2 : Outport  Port=2
  W3 : Outport  Port=3
  wires:
  W6/1(WPos) -> W3/1
  W5/1(WPos) -> W2/1
  W/1(WPos) -> W1/1
  InW3/1 -> W6/1(WIn)
  InW2/1 -> W5/1(WIn)
  InW1/1 -> W/1(WIn)

== system c00010M_harness/M037/S1 ==
  PhyMeasure : Inport
  SensorOut : Outport
  wires:
  PhyMeasure/1 -> SensorOut/1

== system c00010M_harness/M037/S2 ==
  PhyMeasure : Inport
  SensorOut : Outport
  wires:
  PhyMeasure/1 -> SensorOut/1

== system c00010M_harness/M037/S3 ==
  PhyMeasure : Inport
  SensorOut : Outport
  wires:
  PhyMeasure/1 -> SensorOut/1
